simulink model "vnsimulink"  (R2020a)
settings: Solver=ode4  StartTime=0.0  StopTime=20  FixedStep=8e-6  RelTol=1e-3
undefined symbols (not defined in the file or in its folder): D1, Delta, sigbuilder_block
libraries: powerlib x98, powerlib_meascontrol x21, simulink x16
(part 1 of 3)
settings Model: Creator=fengqifan  LastModifiedBy=fengqifan
settings DataIOCC: SaveOutput=off  DSMLogging=off  ReturnWorkspaceOutputs=off
settings DebuggingCC: ArithmeticOperatorsInVariantConditions=warning
settings SFSimCC: CustomCodeUndefinedFunction=UseInterfaceOnly
settings CodeAppCC: StateflowObjectComments=on

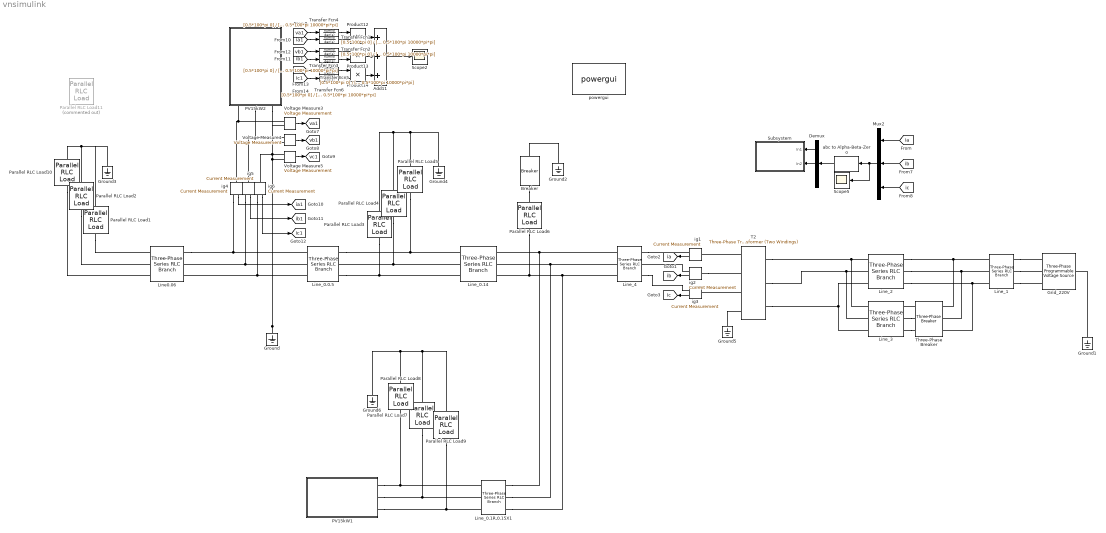
== system vnsimulink ==
  Add11 : Sum  Inputs=+++
  Breaker : powerlib/Elements/Breaker  InitialState=0  SwitchingTimes=[14]  External=off  BreakerResistance=0.001  SnubberResistance=1e6  SnubberCapacitance=inf  Measurements=None  MoreParameters=on  NoBreakLoop=off
  Demux : Demux  Outputs=3
  Grid_220V : powerlib/Electrical Sources/Three-Phase Programmable Voltage Source  PositiveSequence="[400  0 50]"  VariationEntity=None  VariationType=Table of time-amplitude pairs  VariationTypeAlt=Ramp  VariationStep=-0.25  VariationRate=-0  VariationMagnitude=0.3  VariationFrequency=2  VariationTiming=[2 3.5]  VariationPhaseA=on  Amplitudes=[1 0.8 0.6 1.0]  TimeValues=[0 0.5 1 1.5]  HarmonicGeneration=off  HarmonicA=[1 0 -25 0]  HarmonicB=[1 0.3 35 2]  Timing="[2  3]"  BusType=swing  Pref=0  Qref=0  Qmin=-inf  Qmax=inf
  Ground{,1..6} (7 alike) : powerlib/Elements/Ground  LConnTagsString=a
  Line0.06 : powerlib/Elements/Three-Phase Series RLC Branch  LConnTagsString=A|B|C  RConnTagsString=A|B|C  BranchType=RL  Resistance=0.06  Inductance=0.03/(100*pi)  Capacitance=1e-6  Measurements=None
  Line_0.0.5 : powerlib/Elements/Three-Phase Series RLC Branch  LConnTagsString=A|B|C  RConnTagsString=A|B|C  BranchType=RL  Resistance=0.05  Inductance=0.025/(100*pi)  Capacitance=1e-6  Measurements=None
  Line_0.14 : powerlib/Elements/Three-Phase Series RLC Branch  LConnTagsString=A|B|C  RConnTagsString=A|B|C  BranchType=RL  Resistance=0.14  Inductance=0.07/(100*pi)  Capacitance=1e-6  Measurements=None
  Line_0.1R,0.15X1 : powerlib/Elements/Three-Phase Series RLC Branch  LConnTagsString=A|B|C  RConnTagsString=A|B|C  BranchType=RL  Resistance=0.38  Inductance=0.19/(100*pi)  Capacitance=1e-6  Measurements=None
  Line_1 : powerlib/Elements/Three-Phase Series RLC Branch  LConnTagsString=A|B|C  RConnTagsString=A|B|C  BranchType=RL  Resistance=0.03  Inductance=0.02/(100*pi)  Capacitance=1e-6  Measurements=None
  Line_2 : powerlib/Elements/Three-Phase Series RLC Branch  LConnTagsString=A|B|C  RConnTagsString=A|B|C  BranchType=RL  Resistance=0.06  Inductance=0.04/(100*pi)  Capacitance=1e-6  Measurements=None
  Line_3 : powerlib/Elements/Three-Phase Series RLC Branch  LConnTagsString=A|B|C  RConnTagsString=A|B|C  BranchType=RL  Resistance=0.06  Inductance=0.04/(100*pi)  Capacitance=1e-6  Measurements=None
  Line_4 : powerlib/Elements/Three-Phase Series RLC Branch  LConnTagsString=A|B|C  RConnTagsString=A|B|C  BranchType=RL  Resistance=0.08  Inductance=0.085/(100*pi)  Capacitance=1e-6  Measurements=None
  Mux2 : Mux  Inputs=3
  PV15kW1 : Subsystem
  PV15kW2 : Subsystem
  Parallel RLC Load1 : powerlib/Elements/Parallel RLC Load  LConnTagsString=a  RConnTagsString=__new0  NominalVoltage=220  NominalFrequency=50  ActivePower=2e3  InductivePower=1e3  CapacitivePower=0  Setx0=off  InitialVoltage=0  SetiL0=off  InitialCurrent=0  Measurements=None  LoadType=constant Z
      settings: AttributesFormatString=\n  SourceProductBaseCode=PS
  Parallel RLC Load10 : powerlib/Elements/Parallel RLC Load  LConnTagsString=a  RConnTagsString=__new0  NominalVoltage=220  NominalFrequency=50  ActivePower=7e3  InductivePower=2.5e3  CapacitivePower=0  Setx0=off  InitialVoltage=0  SetiL0=off  InitialCurrent=0  Measurements=None  LoadType=constant Z
      settings: AttributesFormatString=\n  SourceProductBaseCode=PS
  Parallel RLC Load11 : powerlib/Elements/Parallel RLC Load  Commented=on  LConnTagsString=a  RConnTagsString=__new0  NominalVoltage=220  NominalFrequency=50  ActivePower=8e3  InductivePower=9e3  CapacitivePower=0  Setx0=off  InitialVoltage=0  SetiL0=off  InitialCurrent=0  Measurements=None  LoadType=constant Z
      settings: AttributesFormatString=\n  SourceProductBaseCode=PS
  Parallel RLC Load2 : powerlib/Elements/Parallel RLC Load  LConnTagsString=a  RConnTagsString=__new0  NominalVoltage=220  NominalFrequency=50  ActivePower=7e3  InductivePower=3.5e3  CapacitivePower=0  Setx0=off  InitialVoltage=0  SetiL0=off  InitialCurrent=0  Measurements=None  LoadType=constant Z
      settings: AttributesFormatString=\n  SourceProductBaseCode=PS
  Parallel RLC Load3 : powerlib/Elements/Parallel RLC Load  LConnTagsString=a  RConnTagsString=__new0  NominalVoltage=220  NominalFrequency=50  ActivePower=6e3  InductivePower=3e3  CapacitivePower=0  Setx0=off  InitialVoltage=0  SetiL0=off  InitialCurrent=0  Measurements=None  LoadType=constant Z
      settings: AttributesFormatString=\n  SourceProductBaseCode=PS
  Parallel RLC Load4 : powerlib/Elements/Parallel RLC Load  LConnTagsString=a  RConnTagsString=__new0  NominalVoltage=220  NominalFrequency=50  ActivePower=5.6e3  InductivePower=2.8e3  CapacitivePower=0  Setx0=off  InitialVoltage=0  SetiL0=off  InitialCurrent=0  Measurements=None  LoadType=constant Z
      settings: AttributesFormatString=\n  SourceProductBaseCode=PS
  Parallel RLC Load5 : powerlib/Elements/Parallel RLC Load  LConnTagsString=a  RConnTagsString=__new0  NominalVoltage=220  NominalFrequency=50  ActivePower=1.6e3  InductivePower=0.8e3  CapacitivePower=0  Setx0=off  InitialVoltage=0  SetiL0=off  InitialCurrent=0  Measurements=None  LoadType=constant Z
      settings: AttributesFormatString=\n  SourceProductBaseCode=PS
  Parallel RLC Load6 : powerlib/Elements/Parallel RLC Load  LConnTagsString=a  RConnTagsString=__new0  NominalVoltage=220  NominalFrequency=50  ActivePower=2e3  InductivePower=1e3  CapacitivePower=0  Setx0=off  InitialVoltage=0  SetiL0=off  InitialCurrent=0  Measurements=None  LoadType=constant Z
      settings: AttributesFormatString=\n  SourceProductBaseCode=PS
  Parallel RLC Load7 : powerlib/Elements/Parallel RLC Load  LConnTagsString=a  RConnTagsString=__new0  NominalVoltage=220  NominalFrequency=50  ActivePower=7.5e3  InductivePower=3e3  CapacitivePower=0  Setx0=off  InitialVoltage=0  SetiL0=off  InitialCurrent=0  Measurements=None  LoadType=constant Z
      settings: AttributesFormatString=\n  SourceProductBaseCode=PS
  Parallel RLC Load8 : powerlib/Elements/Parallel RLC Load  LConnTagsString=a  RConnTagsString=__new0  NominalVoltage=220  NominalFrequency=50  ActivePower=7.5e3  InductivePower=3.5e3  CapacitivePower=0  Setx0=off  InitialVoltage=0  SetiL0=off  InitialCurrent=0  Measurements=None  LoadType=constant Z
      settings: AttributesFormatString=\n  SourceProductBaseCode=PS
  Parallel RLC Load9 : powerlib/Elements/Parallel RLC Load  LConnTagsString=a  RConnTagsString=__new0  NominalVoltage=220  NominalFrequency=50  ActivePower=0.8e3  InductivePower=0.4e3  CapacitivePower=0  Setx0=off  InitialVoltage=0  SetiL0=off  InitialCurrent=0  Measurements=None  LoadType=constant Z
      settings: AttributesFormatString=\n  SourceProductBaseCode=PS
  Product12 : Product
  Product13 : Product
  Product14 : Product
  Scope2 : Scope
  Scope5 : Scope
  Subsystem : Subsystem
  T2 : powerlib/Elements/Three-Phase Transformer (Two Windings)  Winding1Connection=Yn  Winding2Connection=Delta (D1)  CoreType=Three single-phase transformers  SetSaturation=off  Hysteresis=off  DataFile='hysteresis'  SetInitialFlux=off  Measurements=None  UNITS=pu  NominalPower=[10e3 , 50 ]  Winding1=[230 1e-05 1e-06]  Winding2=[220 1e-05 1e-06]  Rm=1  Lm=1  L0=0.5  Saturation=[0 0;0.0024 1.2;0.99998 1.52]  InitialFluxes=[ 0.8 , -0.8 , 0.7 ]  BreakLoop=off  DiscreteSolver=Trapezoidal iterative  DataType=off  TransfoNumber=1
  Three-Phase Breaker : powerlib/Elements/Three-Phase Breaker  InitialState=closed  SwitchA=on  SwitchB=on  SwitchC=on  SwitchTimes=[26]  External=off  BreakerResistance=0.01  SnubberResistance=1e6  SnubberCapacitance=inf  Measurements=None
  Transfer Fcn{1..6} (6 alike) : TransferFcn  Numerator=[0.5*100*pi 0]  Denominator=[1 0.5*100*pi 10000*pi*pi]
  Voltage Measure3 : powerlib/Measurements/Voltage Measurement  PhasorSimulation=off  OutputType=Complex  PSBequivalent=0
  Voltage Measure4 : powerlib/Measurements/Voltage Measurement  PhasorSimulation=off  OutputType=Complex  PSBequivalent=0
  Voltage Measure5 : powerlib/Measurements/Voltage Measurement  PhasorSimulation=off  OutputType=Complex  PSBequivalent=0
  abc to Alpha-Beta-Zero : powerlib_meascontrol/Transformations/abc to Alpha-Beta-Zero
  ig{1..6} (6 alike) : powerlib/Measurements/Current Measurement  PhasorSimulation=off  OutputType=Complex  PSBequivalent=0
  powergui : powerlib/powergui  Priority=1  SimulationMode=Discrete  SampleTime=8e-6  frequency=60  Iterations=50  frequencyindice=0  Pbase=100e6  ErrMax=1e-4  UnitsV=kV  UnitsW=MW  buscounter=0  FunctionMessages=off  echomessages=off  EnableUseOfTLC=off  CurrentSourceSwitches=off  DisableSnubberDevices=off  DisableRonSwitches=off  DisableVfSwitches=off  DisplayEquations=off  AutomaticDiscreteSolvers=off  SolverType=Tustin  Interpol=off  ExternalGateDelay=off  methode=off  Ts=100  x0status=blocks  SPID=on  SwTol=0  HookPort=off  NonlinearTolerance=5e-6  nMaxIteration=100  ContinueOnMaxIteration=off  RestoreLinks=warning  ResistiveCurrentMeasurement=off  Frange=[0:2:500]  Ylog=off  Xlog=on  ShowGrid=off  save=off  variable=ZData  structure=ipv1  ZoomFFT=on  StartTime=0.6  cycles=20  DisplayStyle=1  fundamental=50  FreqAxis=off  MaxFrequency=1000  frequencyindicesteady=1  RmsSteady=1  display=off
  tag scope: ia1=global, ia=global, ib1=global, ib=global, ic1=global, ic=global, va1=global, vb1=global, vc1=global
  wires:
  abc to Alpha-Beta-Zero/1 -> Demux/1
  Demux/2 -> Subsystem/2(In2)
  Demux/1 -> Subsystem/1(In1)
  ig1/1 -> [ia]
  ig3/1 -> [ic]
  ig2/1 -> [ib]
  Mux2/1 -> Scope5/1, abc to Alpha-Beta-Zero/1
  [ib] -> Mux2/2
  [ic] -> Mux2/3
  [ia] -> Mux2/1
  Voltage Measure3/1 -> [va1]
  Voltage Measure4/1 -> [vb1]
  Voltage Measure5/1 -> [vc1]
  ig4/1 -> [ia1]
  ig5/1 -> [ib1]
  ig6/1 -> [ic1]
  [ia1] -> Transfer Fcn1/1
  [va1] -> Transfer Fcn4/1
  [ib1] -> Transfer Fcn3/1
  [vb1] -> Transfer Fcn2/1
  [vc1] -> Transfer Fcn5/1
  [ic1] -> Transfer Fcn6/1
  Product14/1 -> Add11/3
  Product13/1 -> Add11/2
  Product12/1 -> Add11/1
  Add11/1 -> Scope2/1
  Transfer Fcn4/1 -> Product12/1
  Transfer Fcn1/1 -> Product12/2
  Transfer Fcn2/1 -> Product13/1
  Transfer Fcn3/1 -> Product13/2
  Transfer Fcn5/1 -> Product14/1
  Transfer Fcn6/1 -> Product14/2
  connections:
  Line_0.0.5/RConn1 -- Parallel RLC Load5/LConn1 -- Line_0.14/LConn1
  Voltage Measure3/LConn1 -- ig4/LConn1 -- PV15kW2/RConn1
  Parallel RLC Load10/RConn1 -- Parallel RLC Load2/RConn1 -- Ground3/LConn1 -- Parallel RLC Load1/RConn1
  Ground1/LConn1 -- Grid_220V/LConn1
  Line_0.0.5/RConn3 -- Parallel RLC Load3/LConn1 -- Line_0.14/LConn3
  Parallel RLC Load4/LConn1 -- Line_0.14/LConn2 -- Line_0.0.5/RConn2
  Ground/LConn1 -- Voltage Measure5/LConn2 -- Voltage Measure3/LConn2 -- Voltage Measure4/LConn2
  Line_2/RConn3 -- Line_1/LConn3 -- Three-Phase Breaker/RConn3
  Line_2/RConn2 -- Three-Phase Breaker/RConn2 -- Line_1/LConn2
  Parallel RLC Load2/LConn1 -- Line0.06/LConn2
  Parallel RLC Load10/LConn1 -- Line0.06/LConn3
  Line_2/RConn1 -- Line_1/LConn1 -- Three-Phase Breaker/RConn1
  Parallel RLC Load1/LConn1 -- Line0.06/LConn1
  Line_0.0.5/LConn2 -- ig5/RConn1 -- Line0.06/RConn2
  Line_0.0.5/LConn3 -- ig6/RConn1 -- Line0.06/RConn3
  Line_0.1R,0.15X1/RConn2 -- Line_4/LConn2 -- Line_0.14/RConn2
  Line_0.1R,0.15X1/RConn3 -- Line_4/LConn3 -- Parallel RLC Load6/LConn1 -- Line_0.14/RConn3
  Line_3/LConn2 -- T2/RConn2 -- Line_2/LConn2
  Line_3/LConn1 -- T2/RConn1 -- Line_2/LConn1
  Line0.06/RConn1 -- ig4/RConn1 -- Line_0.0.5/LConn1
  PV15kW2/RConn2 -- ig5/LConn1 -- Voltage Measure4/LConn1
  PV15kW2/RConn3 -- ig6/LConn1 -- Voltage Measure5/LConn1
  Parallel RLC Load5/RConn1 -- Ground4/LConn1 -- Parallel RLC Load4/RConn1 -- Parallel RLC Load3/RConn1
  Breaker/LConn1 -- Ground2/LConn1
  Line_3/LConn3 -- Line_2/LConn3 -- T2/RConn3
  Ground5/LConn1 -- T2/LConn4
  T2/LConn1 -- ig1/LConn1
  ig2/LConn1 -- T2/LConn2
  T2/LConn3 -- ig3/LConn1
  Breaker/RConn1 -- Parallel RLC Load6/RConn1
  Line_0.1R,0.15X1/RConn1 -- Line_4/LConn1 -- Line_0.14/RConn1
  Three-Phase Breaker/LConn1 -- Line_3/RConn1
  Line_3/RConn3 -- Three-Phase Breaker/LConn3
  Line_3/RConn2 -- Three-Phase Breaker/LConn2
  Line_1/RConn1 -- Grid_220V/RConn1
  Line_1/RConn2 -- Grid_220V/RConn2
  Line_1/RConn3 -- Grid_220V/RConn3
  Parallel RLC Load8/LConn1 -- PV15kW1/RConn1 -- Line_0.1R,0.15X1/LConn1
  Parallel RLC Load7/LConn1 -- PV15kW1/RConn2 -- Line_0.1R,0.15X1/LConn2
  Parallel RLC Load9/LConn1 -- PV15kW1/RConn3 -- Line_0.1R,0.15X1/LConn3
  Ground6/LConn1 -- Parallel RLC Load9/RConn1 -- Parallel RLC Load7/RConn1 -- Parallel RLC Load8/RConn1
  Line_4/RConn1 -- ig1/RConn1
  ig2/RConn1 -- Line_4/RConn2
  Line_4/RConn3 -- ig3/RConn1

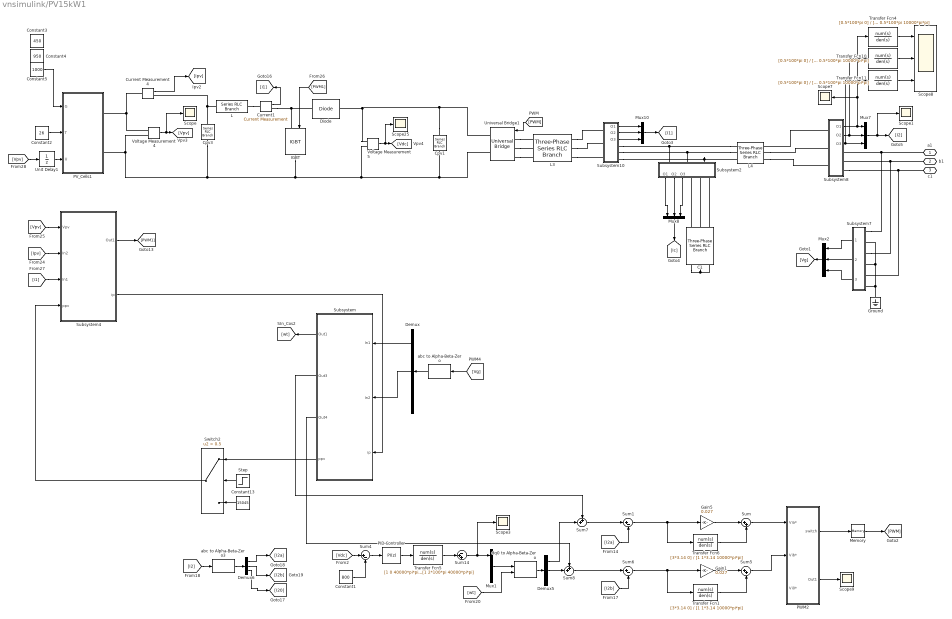
== system vnsimulink/PV15kW1 ==
  C1 : powerlib/Elements/Three-Phase Series RLC Branch  LConnTagsString=A|B|C  RConnTagsString=A|B|C  BranchType=RC  Resistance=13  Inductance=1.5e-3  Capacitance=10e-6  Measurements=None
  Constant1 : Constant  Value=800
  Constant13 : Constant  Value=15045
  Constant2 : Constant  Value=26
  Constant3 : Constant  Value=450
  Constant4 : Constant  Value=950
  Constant5 : Constant  Value=1000
  Cpv1 : powerlib/Elements/Series RLC Branch  LConnTagsString=__new0  RConnTagsString=__new0  BranchType=C  Resistance=0.2  Inductance=0.01e-3  SetiL0=off  InitialCurrent=0  Capacitance=1.6e-3  Setx0=on  InitialVoltage=800  Measurements=None
  Cpv3 : powerlib/Elements/Series RLC Branch  LConnTagsString=__new0  RConnTagsString=__new0  BranchType=C  Resistance=0.001  Inductance=0.01e-3  SetiL0=off  InitialCurrent=0  Capacitance=2e-3  Setx0=on  InitialVoltage=400  Measurements=None
  Current Measurement4 : powerlib/Measurements/Current Measurement  PhasorSimulation=off  OutputType=Complex  PSBequivalent=0
  Current1 : powerlib/Measurements/Current Measurement  PhasorSimulation=off  OutputType=Complex  PSBequivalent=0
  Demux : Demux  Outputs=3
  Demux5 : Demux  Outputs=3
  Demux6 : Demux  Outputs=3
  Diode : powerlib/Power Electronics/Diode  Ron=0.001  Lon=0  Vf=0  IC=0  UseSnubber=0  Rs=inf  Cs=inf  Measurements=off
  Gain1 : Gain  Gain=0.027
  Gain5 : Gain  Gain=0.027
  Ground : powerlib/Elements/Ground  LConnTagsString=a
  IGBT : powerlib/Power Electronics/IGBT  Ron=0.001  Lon=0  Vf=1  Tf=1e-6  Tt=2e-6  IC=0  Rs=1e5  Cs=inf  Measurements=off
  L : powerlib/Elements/Series RLC Branch  LConnTagsString=__new0  RConnTagsString=__new0  BranchType=RL  Resistance=0.02  Inductance=2.5e-3  SetiL0=off  InitialCurrent=0  Capacitance=5e-3  Setx0=off  InitialVoltage=0  Measurements=None
  L3 : powerlib/Elements/Three-Phase Series RLC Branch  LConnTagsString=A|B|C  RConnTagsString=A|B|C  BranchType=RL  Resistance=0.005  Inductance=3.2e-3  Capacitance=1e-6  Measurements=None
  L4 : powerlib/Elements/Three-Phase Series RLC Branch  LConnTagsString=A|B|C  RConnTagsString=A|B|C  BranchType=RL  Resistance=0.005  Inductance=1.6e-3  Capacitance=1e-6  Measurements=None
  Memory : Memory
  Mux{1..2,7..8,10} (5 alike) : Mux  Inputs=3
  PID Controller : simulink/Continuous/PID Controller  Controller=PI  Form=Parallel  TimeDomain=Discrete-time  UseExternalTs=off  SampleTime=2e-4  IntegratorMethod=Forward Euler  FilterMethod=Forward Euler  ControllerParametersSource=internal  P=0.18  I=20  D=0  UseFilter=on  N=100  TunerSelectOption=Transfer Function Based (PID Tuner App)  InitialConditionSource=internal  InitialConditionForIntegrator=0  InitialConditionForFilter=0  DifferentiatorICPrevScaledInput=0  ExternalReset=none  TrackingMode=off  Kt=1  LimitOutput=off  UpperSaturationLimit=inf  LowerSaturationLimit=-inf  LinearizeAsGain=on  AntiWindupMode=none  Kb=1  POutMin=[]  POutMax=[]  IOutMin=[]  IOutMax=[]  DOutMin=[]  DOutMax=[]  NOutMin=[]  NOutMax=[]  SumOutMin=[]  SumOutMax=[]  SaturationOutMin=[]  SaturationOutMax=[]  PParamMin=[]  PParamMax=[]  IParamMin=[]  IParamMax=[]  DParamMin=[]  DParamMax=[]  NParamMin=[]  NParamMax=[]  KbParamMin=[]  KbParamMax=[]  KtParamMin=[]  KtParamMax=[]  KbOutMin=[]  KbOutMax=[]  KtOutMin=[]  KtOutMax=[]  IntegratorOutMin=[]  IntegratorOutMax=[]  FilterOutMin=[]  FilterOutMax=[]  SumI1OutMin=[]  SumI1OutMax=[]  SumI2OutMin=[]  SumI2OutMax=[]  SumI3OutMin=[]  SumI3OutMax=[]  SumI4OutMin=[]  SumI4OutMax=[]  SumDOutMin=[]  SumDOutMax=[]  DifferentiatorOutMin=[]  DifferentiatorOutMax=[]  FilterDiffOutCoefMin=[]  FilterDiffOutCoefMax=[]  ReciprocalOutMin=[]  ReciprocalOutMax=[]  SumDenOutMin=[]  SumDenOutMax=[]  SumNumOutMin=[]  SumNumOutMax=[]  DivideOutMin=[]  DivideOutMax=[]  UdiffTsProdOutMin=[]  UdiffTsProdOutMax=[]  NTsProdOutMin=[]  NTsProdOutMax=[]  UintegralTsProdOutMin=[]  UintegralTsProdOutMax=[]  UngainTsProdOutMin=[]  UngainTsProdOutMax=[]  IntegratorContinuousStateAttributes=''  IntegratorStateMustResolveToSignalObject=off  IntegratorRTWStateStorageClass=Auto  FilterContinuousStateAttributes=''  FilterStateMustResolveToSignalObject=off  FilterRTWStateStorageClass=Auto  ParallelPVariant=InternalParameters  IdealPVariant=Disabled  IVariant=InternalParameters  DVariant=Disabled  IntegratorVariant=Discrete  SatVariant=Disabled  AWVariant=Passthrough  PCopyVariant=Disabled  TRVariant=Disabled  FdbkBlocksVariant=Forward  IdealPFdbkVariant=Disabled  SatFdbkVariant=Disabled  DerivativeFilterVariant=Disabled  NVariant=Disabled  NCopyVariant=Disabled_SignalSpec  FilterICVariant=Disabled  IntegratorICVariant=InternalICs  ExternalResetVariant=Disabled  TRSumVariant=Passthrough  SumFdbkVariant=Disabled  SumVariant=Sum_PI  TsampFilterVariant=InternalTs  TsampNgainVariant=Passthrough  TsampIntegralVariant=Passthrough
  PV_Cells1 : Subsystem  mask{Parallel=5, Series=15}
  PWM2 : Subsystem
  Scope{,1,3,7,9,25} (6 alike) : Scope
  Scope8 : Scope  NumInputPorts=3
  Step : Step  SampleTime=0
  Subsystem : Subsystem
  Subsystem10 : Subsystem
  Subsystem2 : Subsystem
  Subsystem4 : Subsystem
  Subsystem7 : Subsystem
  Subsystem8 : Subsystem
  Sum : Sum  Inputs=|++
  Sum1 : Sum  Inputs=|+-
  Sum14 : Sum  Inputs=-++
  Sum4 : Sum  Inputs=|+-
  Sum5 : Sum  Inputs=|++
  Sum6 : Sum  Inputs=|+-
  Sum7 : Sum  Inputs=++|
  Sum8 : Sum  Inputs=++|
  Switch2 : Switch  Criteria=u2 > Threshold  Threshold=0.5
  Transfer Fcn1 : TransferFcn  Numerator=[3*3.14 0]  Denominator=[1 1*3.14 10000*pi*pi]
  Transfer Fcn10 : TransferFcn  Numerator=[0.5*100*pi 0]  Denominator=[1 0.5*100*pi 10000*pi*pi]
  Transfer Fcn11 : TransferFcn  Numerator=[0.5*100*pi 0]  Denominator=[1 0.5*100*pi 10000*pi*pi]
  Transfer Fcn4 : TransferFcn  Numerator=[0.5*100*pi 0]  Denominator=[1 0.5*100*pi 10000*pi*pi]
  Transfer Fcn5 : TransferFcn  Numerator=[1 0 40000*pi*pi]  Denominator=[1 2*100*pi 40000*pi*pi]
  Transfer Fcn6 : TransferFcn  Numerator=[3*3.14 0]  Denominator=[1 1*3.14 10000*pi*pi]
  Unit Delay1 : UnitDelay  SampleTime=-1  HasFrameUpgradeWarning=on
  Universal Bridge1 : powerlib/Power Electronics/Universal Bridge  Arms=3  SnubberResistance=1e5  SnubberCapacitance=inf  Device=IGBT / Diodes  Ron=0.001  Lon=0  ForwardVoltages="[  0  0  ]"  ForwardVoltage=0  GTOparameters=[ 10e-6 , 20e-6 ]  IGBTparameters=[ 1e-6 , 2e-6 ]  Measurements=None  Measurements_2=None  converterType=Rectifier
  Voltage Measurement4 : powerlib/Measurements/Voltage Measurement  PhasorSimulation=off  OutputType=Complex  PSBequivalent=0
  Voltage Measurement5 : powerlib/Measurements/Voltage Measurement  PhasorSimulation=off  OutputType=Complex  PSBequivalent=0
  abc to Alpha-Beta-Zero : powerlib_meascontrol/Transformations/abc to Alpha-Beta-Zero
  abc to Alpha-Beta-Zero3 : powerlib_meascontrol/Transformations/abc to Alpha-Beta-Zero
  dq0 to Alpha-Beta-Zero : powerlib_meascontrol/Transformations/dq0 to Alpha-Beta-Zero  Alignment=Aligned with phase A axis
      settings: SourceProductBaseCode=PS
  a1 : PMIOPort  Side=Right
  b1 : PMIOPort  Port=2  Side=Right
  c1 : PMIOPort  Port=3  Side=Right
  wires:
  Constant5/1 -> PV_Cells1/1(G)
  Transfer Fcn5/1 -> Sum14/2
  Step/1 -> Switch2/2
  Transfer Fcn11/1 -> Scope8/3
  Transfer Fcn10/1 -> Scope8/2
  Transfer Fcn4/1 -> Scope8/1
  Constant13/1 -> Switch2/3
  Subsystem4/2(ip) -> Subsystem/3(ip)
  Switch2/1 -> Subsystem4/4(ppv)
  Subsystem/4(ppv) -> Switch2/1
  Subsystem/2(Out3) -> Sum7/1
  Subsystem/3(Out4) -> Sum8/1
  [I2] -> abc to Alpha-Beta-Zero3/1
  Demux6/1 -> [I2a]
  abc to Alpha-Beta-Zero3/1 -> Demux6/1
  Demux6/3 -> [I20]
  Demux6/2 -> [I2b]
  Voltage Measurement4/1 -> [Vpv], Scope/1
  [PWM1] -> IGBT/1
  Constant2/1 -> PV_Cells1/2(T)
  [Vpv] -> Unit Delay1/1
  Unit Delay1/1 -> PV_Cells1/3(U)
  Voltage Measurement5/1 -> [Vdc], Scope25/1
  Current1/1 -> [i1]
  Subsystem4/1(Out1) -> [PWM1]
  [Ipv] -> Subsystem4/2(In2)
  [i1] -> Subsystem4/3(In1)
  [Vpv] -> Subsystem4/1(Vpv)
  Current Measurement4/1 -> [Ipv]
  PID Controller/1 -> Transfer Fcn5/1
  Sum14/1 -> Mux1/1, Scope3/1
  Sum8/1 -> Sum6/1
  Demux5/2 -> Sum8/2
  Demux5/1 -> Sum7/2
  Sum7/1 -> Sum1/1
  [I2a] -> Sum1/2
  Transfer Fcn6/1 -> Sum/2
  Sum6/1 -> Gain1/1, Transfer Fcn1/1
  Gain5/1 -> Sum/1
  dq0 to Alpha-Beta-Zero/1 -> Demux5/1
  [wt] -> dq0 to Alpha-Beta-Zero/2
  Sum1/1 -> Gain5/1, Transfer Fcn6/1
  [Vdc] -> Sum4/1
  Mux1/1 -> dq0 to Alpha-Beta-Zero/1
  Sum5/1 -> PWM2/2(Vib*)
  Transfer Fcn1/1 -> Sum5/2
  Constant1/1 -> Sum4/2
  Sum4/1 -> PID Controller/1
  Sum/1 -> PWM2/1(Via*)
  [I2b] -> Sum6/2
  Gain1/1 -> Sum5/1
  abc to Alpha-Beta-Zero/1 -> Demux/1
  Demux/1 -> Subsystem/1(In1)
  [Vg] -> abc to Alpha-Beta-Zero/1
  Demux/2 -> Subsystem/2(In2)
  Subsystem/1(Out1) -> [wt]
  Subsystem7/3(O3) -> Mux2/3
  Subsystem7/2(O2) -> Mux2/2
  Mux8/1 -> [Ic]
  Subsystem10/1(O1) -> Mux10/1
  Subsystem7/1(O1) -> Mux2/1
  Subsystem2/1(O1) -> Mux8/1
  Subsystem8/1(O1) -> Mux7/1, Scope7/1, Transfer Fcn4/1
  Mux2/1 -> [Vg]
  PWM2/1(switch) -> Memory/1
  Subsystem10/3(O3) -> Mux10/3
  Subsystem8/2(O2) -> Transfer Fcn10/1, Mux7/2
  Subsystem8/3(O3) -> Transfer Fcn11/1, Mux7/3
  Subsystem2/3(O3) -> Mux8/3
  Subsystem10/2(O2) -> Mux10/2
  [PWM] -> Universal Bridge1/1
  Mux7/1 -> Scope1/1, [I2]
  PWM2/2(Out1) -> Scope9/1
  Subsystem2/2(O2) -> Mux8/2
  Mux10/1 -> [I1]
  Memory/1 -> [PWM]
  connections:
  Subsystem7/LConn4 -- Subsystem7/LConn6 -- Ground/LConn1 -- Subsystem7/LConn2
  C1/RConn3 -- C1/RConn1 -- C1/RConn2
  Subsystem7/LConn5 -- c1/RConn1 -- Subsystem8/RConn3
  Subsystem8/RConn1 -- a1/RConn1 -- Subsystem7/LConn1
  L/RConn1 -- Current1/LConn1
  L/LConn1 -- Cpv3/LConn1 -- Current Measurement4/RConn1
  Voltage Measurement4/LConn1 -- Current Measurement4/LConn1 -- PV_Cells1/RConn1
  Current1/RConn1 -- Diode/LConn1 -- IGBT/LConn1
  Cpv1/RConn1 -- Universal Bridge1/RConn2 -- Cpv3/RConn1 -- PV_Cells1/RConn2 -- Voltage Measurement4/LConn2 -- IGBT/RConn1 -- Voltage Measurement5/LConn2
  L4/LConn2 -- Subsystem2/LConn2 -- Subsystem10/RConn2
  C1/LConn1 -- Subsystem2/RConn1
  L4/LConn1 -- Subsystem2/LConn1 -- Subsystem10/RConn1
  Subsystem10/RConn3 -- Subsystem2/LConn3 -- L4/LConn3
  Universal Bridge1/LConn3 -- L3/LConn3
  Subsystem8/RConn2 -- b1/RConn1 -- Subsystem7/LConn3
  L4/RConn2 -- Subsystem8/LConn2
  Universal Bridge1/LConn2 -- L3/LConn2
  Cpv1/LConn1 -- Universal Bridge1/RConn1 -- Diode/RConn1 -- Voltage Measurement5/LConn1
  C1/LConn2 -- Subsystem2/RConn2
  L3/RConn3 -- Subsystem10/LConn3
  L3/RConn2 -- Subsystem10/LConn2
  Universal Bridge1/LConn1 -- L3/LConn1
  Subsystem8/LConn1 -- L4/RConn1
  L3/RConn1 -- Subsystem10/LConn1
  L4/RConn3 -- Subsystem8/LConn3
  C1/LConn3 -- Subsystem2/RConn3

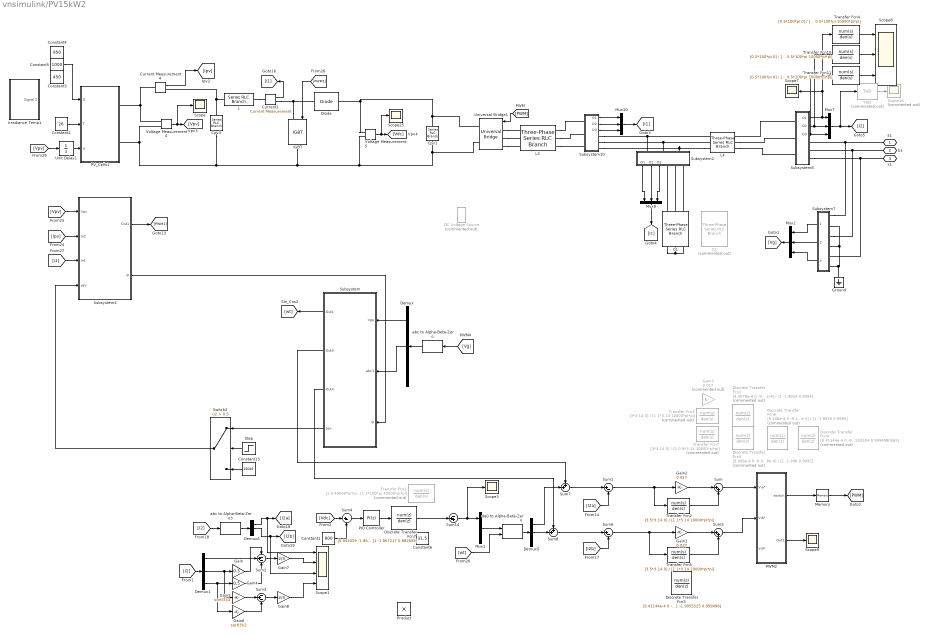
== system vnsimulink/PV15kW2 ==
  C1 : powerlib/Elements/Three-Phase Series RLC Branch  LConnTagsString=A|B|C  RConnTagsString=A|B|C  BranchType=RC  Resistance=13  Inductance=1.5e-3  Capacitance=9e-6  Measurements=None
  C2 : powerlib/Elements/Three-Phase Series RLC Branch  Commented=on  LConnTagsString=A|B|C  RConnTagsString=A|B|C  BranchType=RC  Resistance=13  Inductance=1.5e-3  Capacitance=10e-6  Measurements=None
  Constant1 : Constant  Value=800
  Constant13 : Constant  Value=15045
  Constant2 : Constant  Value=26
  Constant3 : Constant  Value=450
  Constant4 : Constant  Value=950
  Constant5 : Constant  Value=1000
  Constant6 : Constant  Value=31.5
  Cpv1 : powerlib/Elements/Series RLC Branch  LConnTagsString=__new0  RConnTagsString=__new0  BranchType=C  Resistance=0.2  Inductance=0.01e-3  SetiL0=off  InitialCurrent=0  Capacitance=1.6e-3  Setx0=on  InitialVoltage=800  Measurements=None
  Cpv3 : powerlib/Elements/Series RLC Branch  LConnTagsString=__new0  RConnTagsString=__new0  BranchType=C  Resistance=0.001  Inductance=0.01e-3  SetiL0=off  InitialCurrent=0  Capacitance=2e-3  Setx0=on  InitialVoltage=400  Measurements=None
  Current Measurement4 : powerlib/Measurements/Current Measurement  PhasorSimulation=off  OutputType=Complex  PSBequivalent=0
  Current1 : powerlib/Measurements/Current Measurement  PhasorSimulation=off  OutputType=Complex  PSBequivalent=0
  DC Voltage Source : powerlib/Electrical Sources/DC Voltage Source  Commented=on  Amplitude=800  Measurements=None
  Demux{,1,5..6} (4 alike) : Demux  Outputs=3
  Diode : powerlib/Power Electronics/Diode  Ron=0.001  Lon=0  Vf=0  IC=0  UseSnubber=0  Rs=inf  Cs=inf  Measurements=off
  Discrete Transfer Fcn2 : DiscreteTransferFcn  Commented=on  Numerator=[9.4078e-4 0 -9.4078e-4]  Denominator=[1 -1.9954 0.9994]  SampleTime=2e-4
  Discrete Transfer Fcn3 : DiscreteTransferFcn  Numerator=[9.41144e-4 0 -9.41144e-4]  Denominator=[1 -1.9955525 0.999498]  SampleTime=2e-4
  Discrete Transfer Fcn4 : DiscreteTransferFcn  Commented=on  Numerator=[9.41144e-4 0 -9.41144e-4]  Denominator=[1 -1.995552504 0.9994980565]  SampleTime=2e-4
  Discrete Transfer Fcn5 : DiscreteTransferFcn  Commented=on  Numerator=[9.408e-4 0 -9.408e-4]  Denominator=[1 -1.996 0.9995]  SampleTime=2e-4
  Discrete Transfer Fcn6 : DiscreteTransferFcn  Commented=on  Numerator=[9.408e-4 0 -9.408e-4]  Denominator=[1 -1.9956 0.9995]  SampleTime=2e-4
  Discrete Transfer Fcn7 : DiscreteTransferFcn  Numerator=[0.941029 -1.867217 0.941029]  Denominator=[1 -1.867217 0.882058]  SampleTime=2e-4
  Gain : Gain  Gain=0.5
  Gain1 : Gain  Gain=0.027
  Gain2 : Gain  Gain=0.027
  Gain3 : Gain  Commented=on  Gain=0.027
  Gain4 : Gain  Gain=0.5
  Gain5 : Gain  Gain=sqrt(3)/2
  Gain6 : Gain  Gain=sqrt(3)/2
  Gain7 : Gain  Gain=2/3
  Gain8 : Gain  Gain=2/3
  Ground : powerlib/Elements/Ground  LConnTagsString=a
  IGBT : powerlib/Power Electronics/IGBT  Ron=0.001  Lon=0  Vf=1  Tf=1e-6  Tt=2e-6  IC=0  Rs=1e5  Cs=inf  Measurements=off
  Irradiance Temp1 : Subsystem  Tag=STV Subsys  LoadFcn=sigbuilder_block('load');  StartFcn=sigbuilder_block('start');  StopFcn=sigbuilder_block('stop');  ClipboardFcn=sigbuilder_block('clipboard');  mask(Sigbuilder block){tuvar=[0:10]}
      mask help: Sigbuilder GUI
      mask init:
      | if ~strcmp(get_param(bdroot(gcbh),'SimulationStatus'),'stopped') tuvar = sigbuilder_block('maskInit'); end
      settings: CopyFcn=sigbuilder_block('copy');  DeleteFcn=sigbuilder_block('delete');  ModelCloseFcn=sigbuilder_block('modelClose');  PreSaveFcn=sigbuilder_block('preSave');  PauseFcn=sigbuilder_block('pause')  ContinueFcn=sigbuilder_block('continue')  NameChangeFcn=sigbuilder_block('namechange');  OpenFcn=sigbuilder_block('open',[201.375 139.5 550.5 395.25 ]);  CloseFcn=sigbuilder_block('close');
      mask Display: plot(0, 0, 100, 100,[2, 2, 32, 32, 2], [68, 8, 8, 68, 68],[32, 2], [38, 38], [32, 19, 2],[53, 60, 44], [32, 17, 17, 2],[16, 16, 31, 31]);txt = getActiveGroup(gcbh);text(2, 100, txt,'verticalAlignment', 'top');
  L : powerlib/Elements/Series RLC Branch  LConnTagsString=__new0  RConnTagsString=__new0  BranchType=RL  Resistance=0.02  Inductance=2.5e-3  SetiL0=off  InitialCurrent=0  Capacitance=5e-3  Setx0=off  InitialVoltage=0  Measurements=None
  L3 : powerlib/Elements/Three-Phase Series RLC Branch  LConnTagsString=A|B|C  RConnTagsString=A|B|C  BranchType=RL  Resistance=0.005  Inductance=3.2e-3  Capacitance=1e-6  Measurements=None
  L4 : powerlib/Elements/Three-Phase Series RLC Branch  LConnTagsString=A|B|C  RConnTagsString=A|B|C  BranchType=RL  Resistance=0.005  Inductance=1.6e-3  Capacitance=1e-6  Measurements=None
  Memory : Memory
  Mux{1..2,7..8,10} (5 alike) : Mux  Inputs=3
  PID Controller : simulink/Continuous/PID Controller  Controller=PI  Form=Parallel  TimeDomain=Discrete-time  UseExternalTs=off  SampleTime=2e-4  IntegratorMethod=Forward Euler  FilterMethod=Forward Euler  ControllerParametersSource=internal  P=0.15  I=20  D=0  UseFilter=on  N=100  TunerSelectOption=Transfer Function Based (PID Tuner App)  InitialConditionSource=internal  InitialConditionForIntegrator=0  InitialConditionForFilter=0  DifferentiatorICPrevScaledInput=0  ExternalReset=none  TrackingMode=off  Kt=1  LimitOutput=off  UpperSaturationLimit=inf  LowerSaturationLimit=-inf  LinearizeAsGain=on  AntiWindupMode=none  Kb=1  POutMin=[]  POutMax=[]  IOutMin=[]  IOutMax=[]  DOutMin=[]  DOutMax=[]  NOutMin=[]  NOutMax=[]  SumOutMin=[]  SumOutMax=[]  SaturationOutMin=[]  SaturationOutMax=[]  PParamMin=[]  PParamMax=[]  IParamMin=[]  IParamMax=[]  DParamMin=[]  DParamMax=[]  NParamMin=[]  NParamMax=[]  KbParamMin=[]  KbParamMax=[]  KtParamMin=[]  KtParamMax=[]  KbOutMin=[]  KbOutMax=[]  KtOutMin=[]  KtOutMax=[]  IntegratorOutMin=[]  IntegratorOutMax=[]  FilterOutMin=[]  FilterOutMax=[]  SumI1OutMin=[]  SumI1OutMax=[]  SumI2OutMin=[]  SumI2OutMax=[]  SumI3OutMin=[]  SumI3OutMax=[]  SumI4OutMin=[]  SumI4OutMax=[]  SumDOutMin=[]  SumDOutMax=[]  DifferentiatorOutMin=[]  DifferentiatorOutMax=[]  FilterDiffOutCoefMin=[]  FilterDiffOutCoefMax=[]  ReciprocalOutMin=[]  ReciprocalOutMax=[]  SumDenOutMin=[]  SumDenOutMax=[]  SumNumOutMin=[]  SumNumOutMax=[]  DivideOutMin=[]  DivideOutMax=[]  UdiffTsProdOutMin=[]  UdiffTsProdOutMax=[]  NTsProdOutMin=[]  NTsProdOutMax=[]  UintegralTsProdOutMin=[]  UintegralTsProdOutMax=[]  UngainTsProdOutMin=[]  UngainTsProdOutMax=[]  IntegratorContinuousStateAttributes=''  IntegratorStateMustResolveToSignalObject=off  IntegratorRTWStateStorageClass=Auto  FilterContinuousStateAttributes=''  FilterStateMustResolveToSignalObject=off  FilterRTWStateStorageClass=Auto  ParallelPVariant=InternalParameters  IdealPVariant=Disabled  IVariant=InternalParameters  DVariant=Disabled  IntegratorVariant=Discrete  SatVariant=Disabled  AWVariant=Passthrough  PCopyVariant=Disabled  TRVariant=Disabled  FdbkBlocksVariant=Forward  IdealPFdbkVariant=Disabled  SatFdbkVariant=Disabled  DerivativeFilterVariant=Disabled  NVariant=Disabled  NCopyVariant=Disabled_SignalSpec  FilterICVariant=Disabled  IntegratorICVariant=InternalICs  ExternalResetVariant=Disabled  TRSumVariant=Passthrough  SumFdbkVariant=Disabled  SumVariant=Sum_PI  TsampFilterVariant=InternalTs  TsampNgainVariant=Passthrough  TsampIntegralVariant=Passthrough
  PV_Cells1 : Subsystem  mask{Parallel=5, Series=15}
  PWM2 : Subsystem
  Product : Product
  Scope{,3,7,9,25} (5 alike) : Scope
  Scope1 : Scope  NumInputPorts=4
  Scope16 : Scope  Commented=on
  Scope8 : Scope  NumInputPorts=3
  Step : Step  SampleTime=0
  Subsystem : Subsystem
  Subsystem10 : Subsystem
  Subsystem2 : Subsystem
  Subsystem4 : Subsystem
  Subsystem7 : Subsystem
  Subsystem8 : Subsystem
  Sum : Sum  Inputs=|++
  Sum1 : Sum  Inputs=|+-
  Sum14 : Sum  Inputs=-++
  Sum2 : Sum  Inputs=-+-
  Sum3 : Sum  Inputs=-+-
  Sum4 : Sum  Inputs=|+-
  Sum5 : Sum  Inputs=|++
  Sum6 : Sum  Inputs=|+-
  Sum7 : Sum  Inputs=++|
  Sum8 : Sum  Inputs=++|
  Switch2 : Switch  Criteria=u2 > Threshold  Threshold=0.5
  THD : powerlib_meascontrol/Measurements/THD  Commented=on  Freq=50  Ts=0
  Transfer Fcn1 : TransferFcn  Commented=on  Numerator=[1 0 40000*pi*pi]  Denominator=[1 2*100*pi 40000*pi*pi]
  Transfer Fcn10 : TransferFcn  Numerator=[0.5*100*pi 0]  Denominator=[1 0.5*100*pi 10000*pi*pi]
  Transfer Fcn11 : TransferFcn  Numerator=[0.5*100*pi 0]  Denominator=[1 0.5*100*pi 10000*pi*pi]
  Transfer Fcn2 : TransferFcn  Numerator=[3.5*3.14 0]  Denominator=[1 1*3.14 10000*pi*pi]
  Transfer Fcn3 : TransferFcn  Commented=on  Numerator=[3*3.14 0]  Denominator=[1 1*3.14 10000*pi*pi]
  Transfer Fcn4 : TransferFcn  Numerator=[0.5*100*pi 0]  Denominator=[1 0.5*100*pi 10000*pi*pi]
  Transfer Fcn5 : TransferFcn  Numerator=[3.5*3.14 0]  Denominator=[1 1*3.14 10000*pi*pi]
  Transfer Fcn7 : TransferFcn  Commented=on  Numerator=[3*3.14 0]  Denominator=[1 0.8*3.14 10000*pi*pi]
  Unit Delay1 : UnitDelay  SampleTime=-1  HasFrameUpgradeWarning=on
  Universal Bridge1 : powerlib/Power Electronics/Universal Bridge  Arms=3  SnubberResistance=1e5  SnubberCapacitance=inf  Device=IGBT / Diodes  Ron=0.001  Lon=0  ForwardVoltages="[  0  0  ]"  ForwardVoltage=0  GTOparameters=[ 10e-6 , 20e-6 ]  IGBTparameters=[ 1e-6 , 2e-6 ]  Measurements=None  Measurements_2=None  converterType=Rectifier
  Voltage Measurement4 : powerlib/Measurements/Voltage Measurement  PhasorSimulation=off  OutputType=Complex  PSBequivalent=0
  Voltage Measurement5 : powerlib/Measurements/Voltage Measurement  PhasorSimulation=off  OutputType=Complex  PSBequivalent=0
  abc to Alpha-Beta-Zero : powerlib_meascontrol/Transformations/abc to Alpha-Beta-Zero
  abc to Alpha-Beta-Zero3 : powerlib_meascontrol/Transformations/abc to Alpha-Beta-Zero
  dq0 to Alpha-Beta-Zero : powerlib_meascontrol/Transformations/dq0 to Alpha-Beta-Zero  Alignment=Aligned with phase A axis
      settings: SourceProductBaseCode=PS
  a1 : PMIOPort  Side=Right
  b1 : PMIOPort  Port=2  Side=Right
  c1 : PMIOPort  Port=3  Side=Right
  wires:
  Memory/1 -> [PWM]
  Mux10/1 -> [I1]
  Subsystem2/2(O2) -> Mux8/2
  PWM2/2(Out1) -> Scope9/1
  Mux7/1 -> [I2], THD/1
  [PWM] -> Universal Bridge1/1
  Subsystem10/2(O2) -> Mux10/2
  Subsystem2/3(O3) -> Mux8/3
  Subsystem8/3(O3) -> Mux7/3, Transfer Fcn11/1
  Subsystem8/2(O2) -> Mux7/2, Transfer Fcn10/1
  Subsystem10/3(O3) -> Mux10/3
  PWM2/1(switch) -> Memory/1
  Mux2/1 -> [Vg]
  Subsystem8/1(O1) -> Transfer Fcn4/1, Scope7/1, Mux7/1
  Subsystem2/1(O1) -> Mux8/1
  Subsystem7/1(O1) -> Mux2/1
  Subsystem10/1(O1) -> Mux10/1
  Mux8/1 -> [Ic]
  Subsystem7/2(O2) -> Mux2/2
  Subsystem7/3(O3) -> Mux2/3
  Subsystem/1(Out1) -> [wt]
  Demux/2 -> Subsystem/2(abc1)
  [Vg] -> abc to Alpha-Beta-Zero/1
  Demux/1 -> Subsystem/1(Vgq)
  abc to Alpha-Beta-Zero/1 -> Demux/1
  Gain1/1 -> Sum5/1
  [I2b] -> Sum6/2
  Sum/1 -> PWM2/1(Via*)
  Sum4/1 -> PID Controller/1
  Constant1/1 -> Sum4/2
  Sum5/1 -> PWM2/2(Vib*)
  Mux1/1 -> dq0 to Alpha-Beta-Zero/1
  [Vdc] -> Sum4/1
  Sum1/1 -> Transfer Fcn2/1, Gain2/1
  [wt] -> dq0 to Alpha-Beta-Zero/2
  dq0 to Alpha-Beta-Zero/1 -> Demux5/1
  Gain2/1 -> Sum/1
  Sum6/1 -> Transfer Fcn5/1, Gain1/1
  [I2a] -> Sum1/2
  Sum7/1 -> Sum1/1
  Demux5/1 -> Sum7/2
  Demux5/2 -> Sum8/2
  Sum8/1 -> Sum6/1
  Sum14/1 -> Scope3/1, Mux1/1
  PID Controller/1 -> Discrete Transfer Fcn7/1
  THD/1 -> Scope16/1
  Current Measurement4/1 -> [Ipv]
  [Vpv] -> Subsystem4/1(Vpv)
  [i1] -> Subsystem4/3(In1)
  [Ipv] -> Subsystem4/2(In2)
  Subsystem4/1(Out1) -> [PWM1]
  Current1/1 -> [i1]
  Voltage Measurement5/1 -> Scope25/1, [Vdc]
  Unit Delay1/1 -> PV_Cells1/3(U)
  [Vpv] -> Unit Delay1/1
  Constant2/1 -> PV_Cells1/2(T)
  [PWM1] -> IGBT/1
  Voltage Measurement4/1 -> Scope/1, [Vpv]
  Demux6/2 -> Scope1/3, [I2b]
  abc to Alpha-Beta-Zero3/1 -> Demux6/1
  Demux6/1 -> Scope1/1, [I2a]
  [I2] -> abc to Alpha-Beta-Zero3/1
  Subsystem/3(Out4) -> Sum8/1
  Subsystem/2(Out3) -> Sum7/1
  Subsystem/4(ppv) -> Switch2/1
  Switch2/1 -> Subsystem4/4(ppv)
  Subsystem4/2(ip) -> Subsystem/3(ip)
  Constant13/1 -> Switch2/3
  Transfer Fcn4/1 -> Scope8/1
  Transfer Fcn10/1 -> Scope8/2
  Transfer Fcn11/1 -> Scope8/3
  Step/1 -> Switch2/2
  Discrete Transfer Fcn7/1 -> Sum14/2
  [I2] -> Demux1/1
  Demux1/1 -> Sum2/2
  Demux1/2 -> Gain5/1, Gain/1
  Gain/1 -> Sum2/1
  Demux1/3 -> Gain6/1, Gain4/1
  Gain4/1 -> Sum2/3
  Gain5/1 -> Sum3/2
  Gain6/1 -> Sum3/3
  Sum2/1 -> Gain7/1
  Sum3/1 -> Gain8/1
  Gain7/1 -> Scope1/2
  Gain8/1 -> Scope1/4
  Transfer Fcn2/1 -> Sum/2
  Transfer Fcn5/1 -> Sum5/2
  Constant5/1 -> PV_Cells1/1(G)
  connections:
  C1/LConn3 -- Subsystem2/RConn3
  L4/RConn3 -- Subsystem8/LConn3
  L3/RConn1 -- Subsystem10/LConn1
  Subsystem8/LConn1 -- L4/RConn1
  Universal Bridge1/LConn1 -- L3/LConn1
  L3/RConn2 -- Subsystem10/LConn2
  L3/RConn3 -- Subsystem10/LConn3
  C1/LConn2 -- Subsystem2/RConn2
  Voltage Measurement5/LConn1 -- Diode/RConn1 -- Universal Bridge1/RConn1 -- Cpv1/LConn1
  Universal Bridge1/LConn2 -- L3/LConn2
  L4/RConn2 -- Subsystem8/LConn2
  Subsystem7/LConn3 -- b1/RConn1 -- Subsystem8/RConn2
  Universal Bridge1/LConn3 -- L3/LConn3
  L4/LConn3 -- Subsystem2/LConn3 -- Subsystem10/RConn3
  Subsystem10/RConn1 -- Subsystem2/LConn1 -- L4/LConn1
  C1/LConn1 -- Subsystem2/RConn1
  Subsystem10/RConn2 -- Subsystem2/LConn2 -- L4/LConn2
  Voltage Measurement5/LConn2 -- IGBT/RConn1 -- Voltage Measurement4/LConn2 -- PV_Cells1/RConn2 -- Cpv3/RConn1 -- Cpv1/RConn1 -- Universal Bridge1/RConn2
  IGBT/LConn1 -- Diode/LConn1 -- Current1/RConn1
  PV_Cells1/RConn1 -- Current Measurement4/LConn1 -- Voltage Measurement4/LConn1
  Current Measurement4/RConn1 -- Cpv3/LConn1 -- L/LConn1
  L/RConn1 -- Current1/LConn1
  Subsystem7/LConn1 -- a1/RConn1 -- Subsystem8/RConn1
  Subsystem8/RConn3 -- c1/RConn1 -- Subsystem7/LConn5
  C1/RConn2 -- C1/RConn1 -- C1/RConn3
  Subsystem7/LConn2 -- Ground/LConn1 -- Subsystem7/LConn6 -- Subsystem7/LConn4

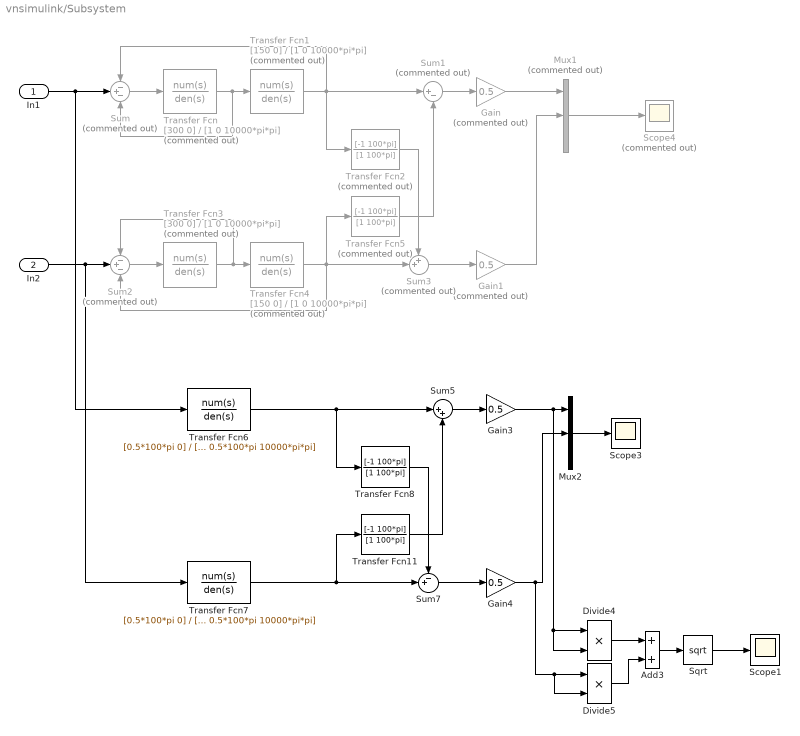
== system vnsimulink/Subsystem ==
  In1 : Inport
  In2 : Inport  Port=2
  Add3 : Sum
  Divide4 : Product  Inputs=**
  Divide5 : Product  Inputs=**
  Gain : Gain  Commented=on  Gain=0.5
  Gain1 : Gain  Commented=on  Gain=0.5
  Gain3 : Gain  Gain=0.5
  Gain4 : Gain  Gain=0.5
  Mux1 : Mux  Commented=on  Inputs=3
  Mux2 : Mux  Inputs=3
  Scope1 : Scope
  Scope3 : Scope
  Scope4 : Scope  Commented=on
  Sqrt : Sqrt  SaturateOnIntegerOverflow=on
  Sum : Sum  Commented=on  Inputs=-+-
  Sum1 : Sum  Commented=on  Inputs=|+-
  Sum2 : Sum  Commented=on  Inputs=-+-
  Sum3 : Sum  Commented=on  Inputs=++|
  Sum5 : Sum  Inputs=|++
  Sum7 : Sum  Inputs=-+|
  Transfer Fcn : TransferFcn  Commented=on  Numerator=[300 0]  Denominator=[1 0 10000*pi*pi]
  Transfer Fcn1 : TransferFcn  Commented=on  Numerator=[150 0]  Denominator=[1 0 10000*pi*pi]
  Transfer Fcn11 : TransferFcn  Numerator=[-1 100*pi]  Denominator=[1 100*pi]
  Transfer Fcn2 : TransferFcn  Commented=on  Numerator=[-1 100*pi]  Denominator=[1 100*pi]
  Transfer Fcn3 : TransferFcn  Commented=on  Numerator=[300 0]  Denominator=[1 0 10000*pi*pi]
  Transfer Fcn4 : TransferFcn  Commented=on  Numerator=[150 0]  Denominator=[1 0 10000*pi*pi]
  Transfer Fcn5 : TransferFcn  Commented=on  Numerator=[-1 100*pi]  Denominator=[1 100*pi]
  Transfer Fcn6 : TransferFcn  Numerator=[0.5*100*pi 0]  Denominator=[1 0.5*100*pi 10000*pi*pi]
  Transfer Fcn7 : TransferFcn  Numerator=[0.5*100*pi 0]  Denominator=[1 0.5*100*pi 10000*pi*pi]
  Transfer Fcn8 : TransferFcn  Numerator=[-1 100*pi]  Denominator=[1 100*pi]
  wires:
  Sum/1 -> Transfer Fcn/1
  Transfer Fcn4/1 -> Transfer Fcn5/1, Sum2/3, Sum3/2
  Sum2/1 -> Transfer Fcn3/1
  Gain1/1 -> Mux1/2
  Transfer Fcn/1 -> Sum/3, Transfer Fcn1/1
  Gain/1 -> Mux1/1
  Transfer Fcn1/1 -> Transfer Fcn2/1, Sum1/1, Sum/1
  Transfer Fcn3/1 -> Transfer Fcn4/1, Sum2/1
  Transfer Fcn2/1 -> Sum3/1
  Transfer Fcn5/1 -> Sum1/2
  Mux1/1 -> Scope4/1
  Sum1/1 -> Gain/1
  Sum3/1 -> Gain1/1
  In2/1 -> Transfer Fcn7/1, Sum2/2
  Sum7/1 -> Gain4/1
  Sum5/1 -> Gain3/1
  Transfer Fcn11/1 -> Sum5/2
  Transfer Fcn8/1 -> Sum7/1
  In1/1 -> Transfer Fcn6/1, Sum/2
  Transfer Fcn6/1 -> Sum5/1, Transfer Fcn8/1
  Transfer Fcn7/1 -> Sum7/2, Transfer Fcn11/1
  Mux2/1 -> Scope3/1
  Sqrt/1 -> Scope1/1
  Gain3/1 -> Divide4/2, Divide4/1, Mux2/1
  Divide5/1 -> Add3/2
  Add3/1 -> Sqrt/1
  Gain4/1 -> Divide5/2, Divide5/1, Mux2/2
  Divide4/1 -> Add3/1

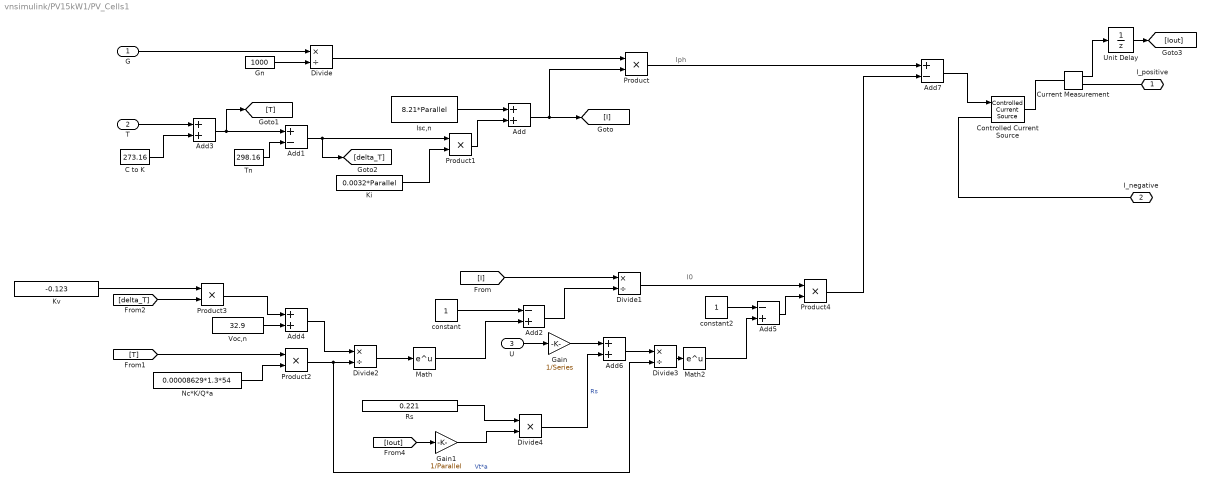
== system vnsimulink/PV15kW1/PV_Cells1 ==
  note: I0
  note: Iph
  G : Inport
  T : Inport  Port=2
  U : Inport  Port=3
  Add{,3..4,6} (4 alike) : Sum
  Add1 : Sum  Inputs=+-
  Add2 : Sum  Inputs=-+
  Add5 : Sum  Inputs=-+
  Add7 : Sum  Inputs=+-
  C to K : Constant  Value=273.16
  Controlled Current Source : powerlib/Electrical Sources/Controlled Current Source  Initialize=on  Source_Type=DC  Amplitude=0  Phase=0  Frequency=0  Measurements=None
  Current Measurement : powerlib/Measurements/Current Measurement  PhasorSimulation=off  OutputType=Complex  PSBequivalent=0
  Divide{,1..3} (4 alike) : Product  Inputs=*/
  Divide4 : Product  Inputs=**
  Gain : Gain  Gain=1/Series
  Gain1 : Gain  Gain=1/Parallel
  Gn : Constant  Value=1000
  Isc,n : Constant  Value=8.21*Parallel
  Ki : Constant  Value=0.0032*Parallel
  Kv : Constant  Value=-0.123
  Math : Math  SignedPower=on  SaturateOnIntegerOverflow=on
  Math2 : Math  SignedPower=on  SaturateOnIntegerOverflow=on
  Nc*K/Q*a : Constant  Value=0.00008629*1.3*54
  Product{,1..4} (5 alike) : Product  RndMeth=Zero
  Rs : Constant  Value=0.221
  Tn : Constant  Value=298.16
  Unit Delay : UnitDelay  SampleTime=-1  HasFrameUpgradeWarning=on
  Voc,n : Constant  Value=32.9
  constant : Constant
  constant2 : Constant
  I_positive : PMIOPort  Tag=PMCPort  Side=Right
  I_negative : PMIOPort  Tag=PMCPort  Port=2  Side=Right
  wires:
  Divide/1 -> Product/1
  Isc,n/1 -> Add/1
  Product1/1 -> Add/2
  Divide2/1 -> Math/1
  Add/1 -> [I], Product/2
  T/1 -> Add3/1
  Add2/1 -> Divide1/2
  Math/1 -> Add2/2
  [I] -> Divide1/1
  Add1/1 -> [delta_T], Product1/1
  Tn/1 -> Add1/2
  Ki/1 -> Product1/2
  Product/1 -> Add7/1
  Nc*K/Q*a/1 -> Product2/2
  Kv/1 -> Product3/1
  Voc,n/1 -> Add4/2
  Current Measurement/1 -> Unit Delay/1
  [T] -> Product2/1
  [delta_T] -> Product3/2
  Add6/1 -> Divide3/1
  U/1 -> Gain/1
  Rs/1 -> Divide4/1
  Divide1/1 -> Product4/1
  Add7/1 -> Controlled Current Source/1
  Product4/1 -> Add7/2
  constant2/1 -> Add5/1
  Add5/1 -> Product4/2
  [Iout] -> Gain1/1
  Math2/1 -> Add5/2
  Divide3/1 -> Math2/1
  C to K/1 -> Add3/2
  Product2/1 -> Divide3/2, Divide2/2  "Vt*a"
  Add4/1 -> Divide2/1
  Product3/1 -> Add4/1
  Gn/1 -> Divide/2
  constant/1 -> Add2/1
  Add3/1 -> [T], Add1/1
  G/1 -> Divide/1
  Unit Delay/1 -> [Iout]
  Gain/1 -> Add6/1
  Gain1/1 -> Divide4/2
  Divide4/1 -> Add6/2  "Rs"
  connections:
  I_negative/RConn1 -- Controlled Current Source/LConn1
  I_positive/RConn1 -- Current Measurement/RConn1
  Controlled Current Source/RConn1 -- Current Measurement/LConn1

== system vnsimulink/PV15kW1/PWM2 ==
  Via* : Inport
  Vib* : Inport  Port=2
  Vi0* : Inport  Port=3
  Alpha-Beta-Zero to abc1 : powerlib_meascontrol/Transformations/Alpha-Beta-Zero to abc
      settings: SourceProductBaseCode=PS
  Bus Creator : BusCreator  Inputs=3
  Demux : Demux  Outputs=3
  Mux1 : Mux  Inputs=3
  PWM : Subsystem
  Transport Delay1 : TransportDelay  Commented=on  DelayTime=1e-4
  switch : Outport  PortDimensions=6
  Out1 : Outport  Port=2
  wires:
  Mux1/1 -> Alpha-Beta-Zero to abc1/1
  Alpha-Beta-Zero to abc1/1 -> Demux/1
  Demux/1 -> Bus Creator/1
  PWM/1(switch) -> switch/1
  Demux/3 -> Bus Creator/3
  Demux/2 -> Bus Creator/2
  Vi0*/1 -> Mux1/3
  Vib*/1 -> Mux1/2
  Via*/1 -> Mux1/1
  Bus Creator/1 -> PWM/1(In1)
  PWM/2(Out1) -> Out1/1

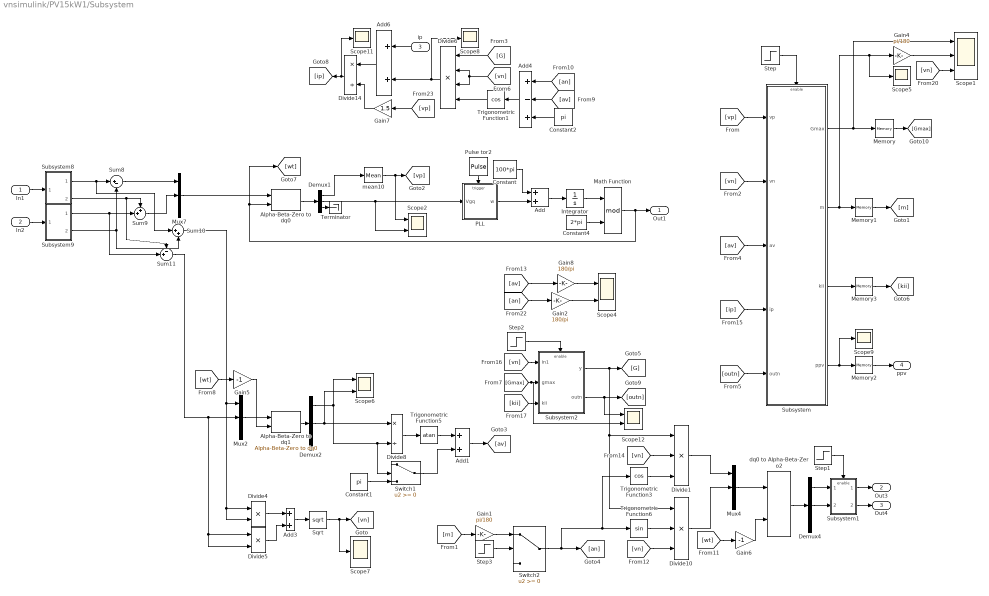
== system vnsimulink/PV15kW1/Subsystem ==
  In1 : Inport
  In2 : Inport  Port=2
  ip : Inport  Port=3
  Add{,1,3,6} (4 alike) : Sum
  Add4 : Sum  Inputs=+-+
  Alpha-Beta-Zero to dq0 : powerlib_meascontrol/Transformations/Alpha-Beta-Zero to dq0  Alignment=Aligned with phase A axis
  Alpha-Beta-Zero to dq1 : powerlib_meascontrol/Transformations/Alpha-Beta-Zero to dq0  Alignment=Aligned with phase A axis
  Constant : Constant  Value=100*pi
  Constant1 : Constant  Value=pi
  Constant2 : Constant  Value=pi
  Constant4 : Constant  Value=2*pi
  Demux1 : Demux  Outputs=3
  Demux2 : Demux  Outputs=3
  Demux4 : Demux  Outputs=3
  Divide1 : Product  Inputs=***
  Divide10 : Product  Inputs=***
  Divide14 : Product  Inputs=*/
  Divide4 : Product  Inputs=**
  Divide5 : Product  Inputs=**
  Divide6 : Product  Inputs=****
  Divide8 : Product  Inputs=*/
  Gain1 : Gain  Gain=pi/180
  Gain2 : Gain  Gain=180/pi
  Gain4 : Gain  Gain=pi/180
  Gain5 : Gain  Gain=-1
  Gain6 : Gain  Gain=-1
  Gain7 : Gain  Gain=1.5
  Gain8 : Gain  Gain=180/pi
  Integrator : Integrator
  Math Function : Math  Operator=mod  SignedPower=on  SaturateOnIntegerOverflow=on
  Memory{,1..3} (4 alike) : Memory
  Mux2 : Mux  Inputs=3
  Mux4 : Mux  Inputs=3
  Mux7 : Mux  Inputs=3
  PLL : Subsystem  TreatAsAtomicUnit=on
  Pulse tor2 : DiscretePulseGenerator  PulseType=Time based  Period=2e-4  PulseWidth=40
  Scope1 : Scope  NumInputPorts=3
  Scope{5,7..9,11} (5 alike) : Scope
  Scope{2,4,6,12} (4 alike) : Scope  NumInputPorts=2
  Sqrt : Sqrt  SaturateOnIntegerOverflow=on
  Step : Step  Time=0.9922  SampleTime=0
  Step1 : Step  SampleTime=0
  Step2 : Step  SampleTime=0
  Step3 : Step  SampleTime=0
  Subsystem : Subsystem
  Subsystem1 : Subsystem
  Subsystem2 : Subsystem
  Subsystem8 : Subsystem
  Subsystem9 : Subsystem
  Sum10 : Sum  Inputs=|++
  Sum11 : Sum  Inputs=-+|
  Sum8 : Sum  Inputs=|+-
  Sum9 : Sum  Inputs=++|
  Switch1 : Switch
  Switch2 : Switch
  Terminator : Terminator
  Trigonometric Function1 : Trigonometry  Operator=cos
  Trigonometric Function3 : Trigonometry  Operator=cos
  Trigonometric Function5 : Trigonometry  Operator=atan
  Trigonometric Function6 : Trigonometry
  dq0 to Alpha-Beta-Zero2 : powerlib_meascontrol/Transformations/dq0 to Alpha-Beta-Zero  Alignment=Aligned with phase A axis
      settings: SourceProductBaseCode=PS
  mean10 : powerlib_meascontrol/Measurements/Mean  Freq=100  Vinit=0  Ts=2e-4
  Out1 : Outport
  Out3 : Outport  Port=2
  Out4 : Outport  Port=3
  ppv : Outport  Port=4
  wires:
  [vn] -> Scope1/3
  Subsystem/3(kii) -> Memory3/1
  [vn] -> Divide1/2
  Memory3/1 -> [kii]
  [kii] -> Subsystem2/3(kii)
  Divide14/1 -> [ip], Scope11/1
  [ip] -> Subsystem/4(ip)
  Constant2/1 -> Add4/3
  [av] -> Gain8/1
  Divide6/1 -> Scope8/1, Add6/2
  [G] -> Divide6/1
  [an] -> Add4/1
  [av] -> Add4/2
  Trigonometric Function1/1 -> Divide6/4
  [vn] -> Divide6/2, Divide6/3
  Add4/1 -> Trigonometric Function1/1
  Switch2/1 -> Trigonometric Function3/1, Trigonometric Function6/1, [an]
  [Gmax] -> Scope12/2, Subsystem2/2(gmax)
  [outn] -> Subsystem/5(outn)
  Demux1/3 -> Terminator/1
  [vp] -> Subsystem/1(vp)
  [m] -> Gain1/1
  Gain4/1 -> Scope1/2
  Memory1/1 -> [m]
  Gain1/1 -> Switch2/1
  Step3/1 -> Switch2/2
  Subsystem/2(m) -> Gain4/1, Scope5/1, Memory1/1
  [an] -> Gain2/1
  Trigonometric Function6/1 -> Divide10/2
  Subsystem2/1(y) -> Divide10/1, Divide1/1, [G]
  Subsystem1/1(Out3) -> Out3/1
  dq0 to Alpha-Beta-Zero2/1 -> Demux4/1
  Mux7/1 -> Alpha-Beta-Zero to dq0/1
  Sum11/1 -> Divide5/1, Divide5/2, Mux2/2
  Sum10/1 -> Mux2/1, Divide4/1, Divide4/2
  Sum9/1 -> Mux7/2
  Sum8/1 -> Mux7/1
  Subsystem8/2(Out2) -> Sum9/1, Sum11/1
  Subsystem9/1(Out1) -> Sum9/2, Sum11/2
  Subsystem9/2(Out2) -> Sum10/2, Sum8/2
  Subsystem8/1(Out1) -> Sum8/1, Sum10/1
  Memory2/1 -> ppv/1
  Gain7/1 -> Divide14/2
  Add6/1 -> Divide14/1
  ip/1 -> Add6/1
  mean10/1 -> [vp], Scope2/1
  [av] -> Subsystem/3(av)
  Demux2/2 -> Divide8/1, Scope6/2
  Demux2/1 -> Divide8/2, Switch1/2, Scope6/1
  [vn] -> Subsystem/2(vn)
  [vp] -> Gain7/1
  Sqrt/1 -> Scope7/1, [vn]
  Switch1/1 -> Add1/2
  Add1/1 -> [av]
  Trigonometric Function5/1 -> Add1/1
  Gain2/1 -> Scope4/2
  Gain8/1 -> Scope4/1
  Memory/1 -> [Gmax]
  Subsystem2/2(outn) -> [outn], Scope12/1
  Demux1/2 -> PLL/1(Vgq), Scope2/2
  Subsystem/4(ppv) -> Scope9/1, Memory2/1
  Step2/1 -> Subsystem2/Enable
  [vn] -> Subsystem2/1(In1)
  Subsystem/1(Gmax) -> Memory/1, Scope1/1
  In1/1 -> Subsystem8/1(In1)
  In2/1 -> Subsystem9/1(In1)
  Gain6/1 -> dq0 to Alpha-Beta-Zero2/2
  Gain5/1 -> Alpha-Beta-Zero to dq1/2
  Subsystem1/2(Out4) -> Out4/1
  Step1/1 -> Subsystem1/Enable
  Demux4/2 -> Subsystem1/2(In3)
  Demux4/1 -> Subsystem1/1(In2)
  Mux4/1 -> dq0 to Alpha-Beta-Zero2/1
  Divide1/1 -> Mux4/1
  Step/1 -> Subsystem/Enable
  [vn] -> Divide10/3
  Trigonometric Function3/1 -> Divide1/3
  [wt] -> Gain6/1
  Divide10/1 -> Mux4/2
  [wt] -> Gain5/1
  Divide5/1 -> Add3/2
  Divide4/1 -> Add3/1
  Add3/1 -> Sqrt/1
  Divide8/1 -> Trigonometric Function5/1
  Constant1/1 -> Switch1/3
  Alpha-Beta-Zero to dq1/1 -> Demux2/1
  Mux2/1 -> Alpha-Beta-Zero to dq1/1
  Integrator/1 -> Math Function/1
  Pulse tor2/1 -> PLL/Trigger
  Constant4/1 -> Math Function/2
  Demux1/1 -> mean10/1
  Alpha-Beta-Zero to dq0/1 -> Demux1/1
  PLL/1(w) -> Add/2
  Constant/1 -> Add/1
  Math Function/1 -> Alpha-Beta-Zero to dq0/2, [wt], Out1/1
  Add/1 -> Integrator/1

== system vnsimulink/PV15kW1/Subsystem10 ==
  Current : powerlib/Measurements/Current Measurement  PhasorSimulation=off  OutputType=Complex  PSBequivalent=0
  Current 2 : powerlib/Measurements/Current Measurement  PhasorSimulation=off  OutputType=Complex  PSBequivalent=0
  Current1 : powerlib/Measurements/Current Measurement  PhasorSimulation=off  OutputType=Complex  PSBequivalent=0
  1 : PMIOPort  Side=Left
  2 : PMIOPort  Port=2  Side=Right
  3 : PMIOPort  Port=3  Side=Left
  4 : PMIOPort  Port=4  Side=Right
  5 : PMIOPort  Port=5  Side=Left
  6 : PMIOPort  Port=6  Side=Right
  O1 : Outport
  O2 : Outport  Port=2
  O3 : Outport  Port=3
  wires:
  Current 2/1 -> O3/1
  Current1/1 -> O2/1
  Current/1 -> O1/1
  connections:
  6/RConn1 -- Current 2/RConn1
  5/RConn1 -- Current 2/LConn1
  4/RConn1 -- Current1/RConn1
  3/RConn1 -- Current1/LConn1
  2/RConn1 -- Current/RConn1
  1/RConn1 -- Current/LConn1
